simulink model "Mo_phong"  (R2016a)
settings: Solver=ode5  SolverMode=SingleTasking  StartTime=0.0  StopTime=9  FixedStep=0.001  RelTol=1e-3
libraries: simulink x5
settings Model: Creator=nguye  LastModifiedBy=nguye
settings DebuggingCC: SFUnexpectedBacktrackingDiag=error  SFNoUnconditionalDefaultTransitionDiag=error
settings SFSimCC: SimUseLocalCustomCode=on
settings RTWCC: RTWUseLocalCustomCode=on
settings GRTTargetCC: TargetLangStandard=C99 (ISO)  GeneratePreprocessorConditionals=Use local settings
settings ConfigComp: CovMetricSettings=dwe  CovHtmlReporting=off  CovSaveCumulativeToWorkspaceVar=off  CovSaveSingleToWorkspaceVar=off  CovExternalEMLEnable=on

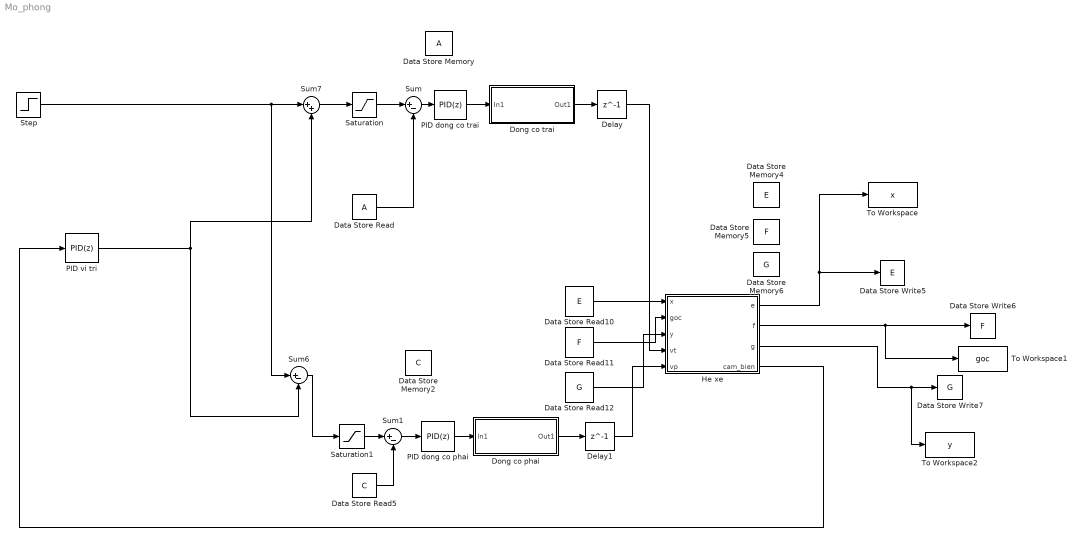
== system Mo_phong ==
  Data Store Memory : DataStoreMemory  ReadBeforeWriteMsg=warning  WriteAfterWriteMsg=warning  WriteAfterReadMsg=warning  ShowAdditionalParam=off
  Data Store Memory2 : DataStoreMemory  DataStoreName=C  ReadBeforeWriteMsg=warning  WriteAfterWriteMsg=warning  WriteAfterReadMsg=warning  ShowAdditionalParam=off
  Data Store Memory4 : DataStoreMemory  DataStoreName=E  ReadBeforeWriteMsg=warning  WriteAfterWriteMsg=warning  WriteAfterReadMsg=warning  ShowAdditionalParam=off
  Data Store Memory5 : DataStoreMemory  DataStoreName=F  ReadBeforeWriteMsg=warning  WriteAfterWriteMsg=warning  WriteAfterReadMsg=warning  ShowAdditionalParam=off
  Data Store Memory6 : DataStoreMemory  DataStoreName=G  ReadBeforeWriteMsg=warning  WriteAfterWriteMsg=warning  WriteAfterReadMsg=warning  ShowAdditionalParam=off
  Data Store Read : DataStoreRead
  Data Store Read10 : DataStoreRead  DataStoreName=E
  Data Store Read11 : DataStoreRead  DataStoreName=F
  Data Store Read12 : DataStoreRead  DataStoreName=G
  Data Store Read5 : DataStoreRead  DataStoreName=C
  Data Store Write5 : DataStoreWrite  DataStoreName=E
  Data Store Write6 : DataStoreWrite  DataStoreName=F
  Data Store Write7 : DataStoreWrite  DataStoreName=G
  Delay : Delay  DelayLength=1  InitialCondition=0
  Delay1 : Delay  DelayLength=1  InitialCondition=0
  Dong co phai : Subsystem
  Dong co trai : Subsystem
  He xe : MATLAB Function  TreatAsAtomicUnit=on
  PID dong co phai : simulink/Continuous/PID Controller  Controller=PID  Form=Parallel  TimeDomain=Discrete-time  SampleTime=0.001  IntegratorMethod=Forward Euler  FilterMethod=Forward Euler  ControllerParametersSource=internal  P=0.25  I=8  D=0.0  UseFilter=off  N=0.08  InitialConditionSource=internal  InitialConditionForIntegrator=0  InitialConditionForFilter=0  DifferentiatorICPrevScaledInput=0  ExternalReset=none  TrackingMode=off  Kt=1  LimitOutput=on  UpperSaturationLimit=100  LowerSaturationLimit=-100  LinearizeAsGain=off  AntiWindupMode=none  Kb=1  POutMin=[]  POutMax=[]  IOutMin=[]  IOutMax=[]  DOutMin=[]  DOutMax=[]  NOutMin=[]  NOutMax=[]  SumOutMin=[]  SumOutMax=[]  SaturationOutMin=[]  SaturationOutMax=[]  PParamMin=[]  PParamMax=[]  IParamMin=[]  IParamMax=[]  DParamMin=[]  DParamMax=[]  NParamMin=[]  NParamMax=[]  KbParamMin=[]  KbParamMax=[]  KtParamMin=[]  KtParamMax=[]  KbOutMin=[]  KbOutMax=[]  KtOutMin=[]  KtOutMax=[]  IntegratorOutMin=[]  IntegratorOutMax=[]  FilterOutMin=[]  FilterOutMax=[]  SumI1OutMin=[]  SumI1OutMax=[]  SumI2OutMin=[]  SumI2OutMax=[]  SumI3OutMin=[]  SumI3OutMax=[]  SumDOutMin=[]  SumDOutMax=[]  DifferentiatorOutMin=[]  DifferentiatorOutMax=[]  IntegratorContinuousStateAttributes=''  IntegratorStateMustResolveToSignalObject=off  IntegratorRTWStateStorageClass=Auto  FilterContinuousStateAttributes=''  FilterStateMustResolveToSignalObject=off  FilterRTWStateStorageClass=Auto
  PID dong co trai : simulink/Continuous/PID Controller  Controller=PID  Form=Parallel  TimeDomain=Discrete-time  SampleTime=0.001  IntegratorMethod=Forward Euler  FilterMethod=Forward Euler  ControllerParametersSource=internal  P=0.25  I=7.5  D=0.0  UseFilter=off  N=0.08  InitialConditionSource=internal  InitialConditionForIntegrator=0  InitialConditionForFilter=0  DifferentiatorICPrevScaledInput=0  ExternalReset=none  TrackingMode=off  Kt=1  LimitOutput=on  UpperSaturationLimit=100  LowerSaturationLimit=-100  LinearizeAsGain=off  AntiWindupMode=none  Kb=1  POutMin=[]  POutMax=[]  IOutMin=[]  IOutMax=[]  DOutMin=[]  DOutMax=[]  NOutMin=[]  NOutMax=[]  SumOutMin=[]  SumOutMax=[]  SaturationOutMin=[]  SaturationOutMax=[]  PParamMin=[]  PParamMax=[]  IParamMin=[]  IParamMax=[]  DParamMin=[]  DParamMax=[]  NParamMin=[]  NParamMax=[]  KbParamMin=[]  KbParamMax=[]  KtParamMin=[]  KtParamMax=[]  KbOutMin=[]  KbOutMax=[]  KtOutMin=[]  KtOutMax=[]  IntegratorOutMin=[]  IntegratorOutMax=[]  FilterOutMin=[]  FilterOutMax=[]  SumI1OutMin=[]  SumI1OutMax=[]  SumI2OutMin=[]  SumI2OutMax=[]  SumI3OutMin=[]  SumI3OutMax=[]  SumDOutMin=[]  SumDOutMax=[]  DifferentiatorOutMin=[]  DifferentiatorOutMax=[]  IntegratorContinuousStateAttributes=''  IntegratorStateMustResolveToSignalObject=off  IntegratorRTWStateStorageClass=Auto  FilterContinuousStateAttributes=''  FilterStateMustResolveToSignalObject=off  FilterRTWStateStorageClass=Auto
  PID vi tri : simulink/Continuous/PID Controller  Controller=PID  Form=Parallel  TimeDomain=Discrete-time  SampleTime=-1  IntegratorMethod=Forward Euler  FilterMethod=Forward Euler  ControllerParametersSource=internal  P=10  I=0  D=2  UseFilter=on  N=1  InitialConditionSource=internal  InitialConditionForIntegrator=0  InitialConditionForFilter=0  DifferentiatorICPrevScaledInput=0  ExternalReset=none  TrackingMode=off  Kt=1  LimitOutput=off  UpperSaturationLimit=inf  LowerSaturationLimit=-inf  LinearizeAsGain=off  AntiWindupMode=none  Kb=1  POutMin=[]  POutMax=[]  IOutMin=[]  IOutMax=[]  DOutMin=[]  DOutMax=[]  NOutMin=[]  NOutMax=[]  SumOutMin=[]  SumOutMax=[]  SaturationOutMin=[]  SaturationOutMax=[]  PParamMin=[]  PParamMax=[]  IParamMin=[]  IParamMax=[]  DParamMin=[]  DParamMax=[]  NParamMin=[]  NParamMax=[]  KbParamMin=[]  KbParamMax=[]  KtParamMin=[]  KtParamMax=[]  KbOutMin=[]  KbOutMax=[]  KtOutMin=[]  KtOutMax=[]  IntegratorOutMin=[]  IntegratorOutMax=[]  FilterOutMin=[]  FilterOutMax=[]  SumI1OutMin=[]  SumI1OutMax=[]  SumI2OutMin=[]  SumI2OutMax=[]  SumI3OutMin=[]  SumI3OutMax=[]  SumDOutMin=[]  SumDOutMax=[]  DifferentiatorOutMin=[]  DifferentiatorOutMax=[]  IntegratorContinuousStateAttributes=''  IntegratorStateMustResolveToSignalObject=off  IntegratorRTWStateStorageClass=Auto  FilterContinuousStateAttributes=''  FilterStateMustResolveToSignalObject=off  FilterRTWStateStorageClass=Auto
  Saturation : Saturate  UpperLimit=292  LowerLimit=25
  Saturation1 : Saturate  UpperLimit=258  LowerLimit=25
  Step : Step  Time=0  After=100
  Sum : Sum  Inputs=|+-
  Sum1 : Sum  Inputs=|+-
  Sum6 : Sum  Inputs=|+-
  Sum7 : Sum  Inputs=|++
  To Workspace : ToWorkspace  VariableName=x  SampleTime=-1
      settings: Save2DSignal=2-D array (concatenate along first dimension)
  To Workspace1 : ToWorkspace  VariableName=goc  SampleTime=-1
      settings: Save2DSignal=2-D array (concatenate along first dimension)
  To Workspace2 : ToWorkspace  VariableName=y  SampleTime=-1
      settings: Save2DSignal=2-D array (concatenate along first dimension)
  wires:
  Step/1 -> Sum6/1, Sum7/1
  Data Store Read/1 -> Sum/2
  Sum/1 -> PID dong co trai/1
  Sum1/1 -> PID dong co phai/1
  Data Store Read5/1 -> Sum1/2
  Sum6/1 -> Saturation1/1
  Sum7/1 -> Saturation/1
  Saturation/1 -> Sum/1
  Saturation1/1 -> Sum1/1
  Delay/1 -> He xe/4(vt)
  Delay1/1 -> He xe/5(vp)
  Data Store Read10/1 -> He xe/1(x)
  Data Store Read11/1 -> He xe/2(goc)
  Data Store Read12/1 -> He xe/3(y)
  He xe/1(e) -> To Workspace/1, Data Store Write5/1
  He xe/2(f) -> Data Store Write6/1, To Workspace1/1
  He xe/3(g) -> Data Store Write7/1, To Workspace2/1
  He xe/4(cam_bien) -> PID vi tri/1
  PID vi tri/1 -> Sum7/2, Sum6/2
  PID dong co trai/1 -> Dong co trai/1(In1)
  Dong co trai/1(Out1) -> Delay/1
  PID dong co phai/1 -> Dong co phai/1(In1)
  Dong co phai/1(Out1) -> Delay1/1

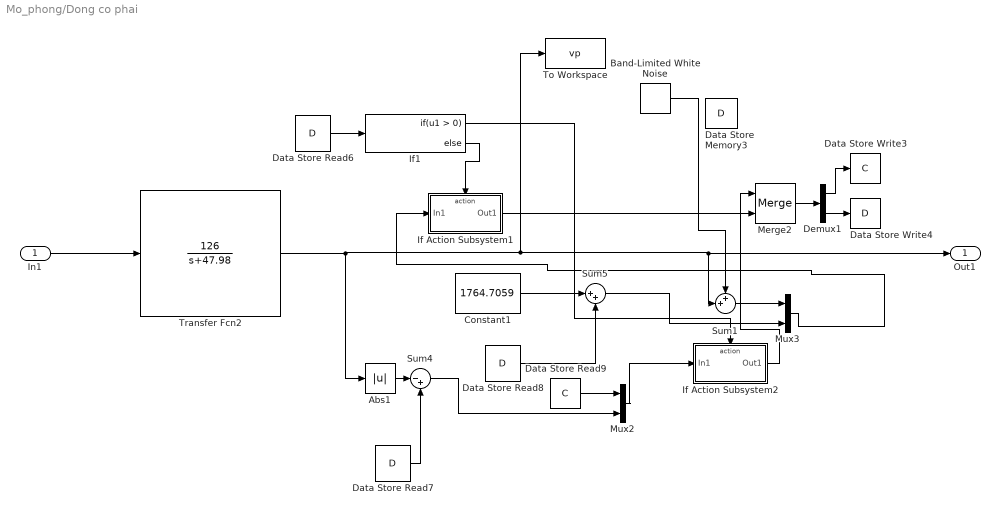
== system Mo_phong/Dong co phai ==
  In1 : Inport
  Abs1 : Abs
  Band-Limited White Noise : simulink/Sources/Band-Limited White Noise  Cov=[0.005]  Ts=0.001  seed=[23341]
  Constant1 : Constant  Value=1764.7059
  Data Store Memory3 : DataStoreMemory  DataStoreName=D  ReadBeforeWriteMsg=warning  WriteAfterWriteMsg=warning  WriteAfterReadMsg=warning  InitialValue=1764.7059  ShowAdditionalParam=off
  Data Store Read6 : DataStoreRead  DataStoreName=D
  Data Store Read7 : DataStoreRead  DataStoreName=D
  Data Store Read8 : DataStoreRead  DataStoreName=D
  Data Store Read9 : DataStoreRead  DataStoreName=C
  Data Store Write3 : DataStoreWrite  DataStoreName=C
  Data Store Write4 : DataStoreWrite  DataStoreName=D
  Demux1 : Demux  Outputs=2
  If Action Subsystem1 : Subsystem  TreatAsAtomicUnit=on
  If Action Subsystem2 : Subsystem  TreatAsAtomicUnit=on
  If1 : If
  Merge2 : Merge
  Mux2 : Mux  Inputs=2
  Mux3 : Mux  Inputs=2
  Sum1 : Sum  Inputs=++|
  Sum4 : Sum  Inputs=|-+
  Sum5 : Sum  Inputs=|++
  To Workspace : ToWorkspace  VariableName=vp  SampleTime=-1
      settings: Save2DSignal=2-D array (concatenate along first dimension)
  Transfer Fcn2 : TransferFcn  Numerator=[126]  Denominator=[1 47.98]
  Out1 : Outport
  wires:
  Sum4/1 -> Mux2/2
  Transfer Fcn2/1 -> To Workspace/1, Sum1/2, Out1/1, Abs1/1
  Data Store Read6/1 -> If1/1
  If Action Subsystem1/1(Out1) -> Merge2/2
  Data Store Read8/1 -> Sum5/2
  Data Store Read7/1 -> Sum4/2
  Sum5/1 -> Mux3/2
  If1/1 -> If Action Subsystem2/Action
  Abs1/1 -> Sum4/1
  If1/2 -> If Action Subsystem1/Action
  Constant1/1 -> Sum5/1
  Mux2/1 -> If Action Subsystem2/1(In1)
  Demux1/2 -> Data Store Write4/1
  Mux3/1 -> If Action Subsystem1/1(In1)
  In1/1 -> Transfer Fcn2/1
  Data Store Read9/1 -> Mux2/1
  Merge2/1 -> Demux1/1
  If Action Subsystem2/1(Out1) -> Merge2/1
  Demux1/1 -> Data Store Write3/1
  Sum1/1 -> Mux3/1
  Band-Limited White Noise/1 -> Sum1/1

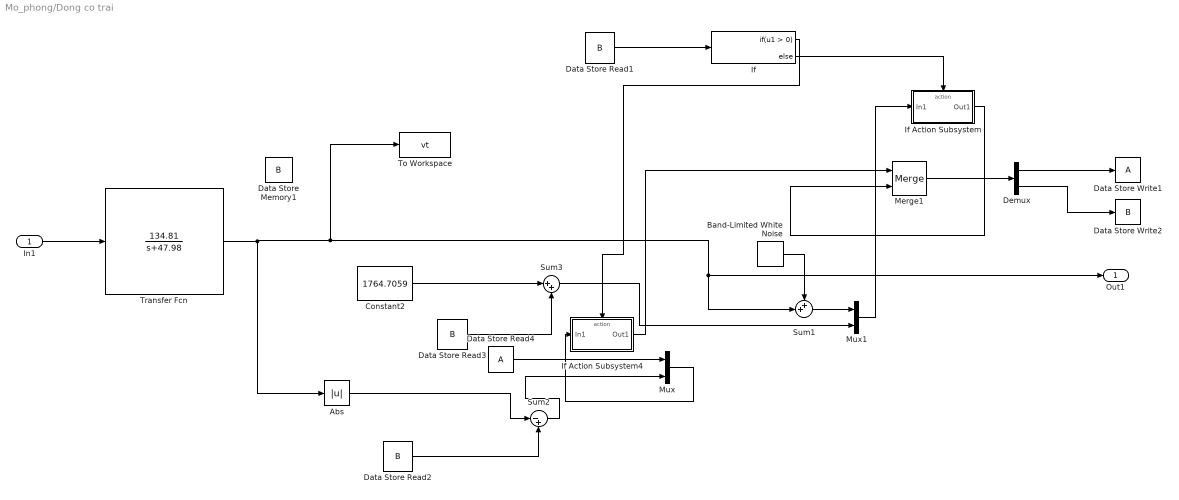
== system Mo_phong/Dong co trai ==
  In1 : Inport
  Abs : Abs
  Band-Limited White Noise : simulink/Sources/Band-Limited White Noise  Cov=[0.005]  Ts=0.001  seed=[23341]
  Constant2 : Constant  Value=1764.7059
  Data Store Memory1 : DataStoreMemory  DataStoreName=B  ReadBeforeWriteMsg=warning  WriteAfterWriteMsg=warning  WriteAfterReadMsg=warning  InitialValue=1764.7059  ShowAdditionalParam=off
  Data Store Read1 : DataStoreRead  DataStoreName=B
  Data Store Read2 : DataStoreRead  DataStoreName=B
  Data Store Read3 : DataStoreRead  DataStoreName=B
  Data Store Read4 : DataStoreRead
  Data Store Write1 : DataStoreWrite
  Data Store Write2 : DataStoreWrite  DataStoreName=B
  Demux : Demux  Outputs=2
  If : If
  If Action Subsystem : Subsystem  TreatAsAtomicUnit=on
  If Action Subsystem4 : Subsystem  TreatAsAtomicUnit=on
  Merge1 : Merge
  Mux : Mux  Inputs=2
  Mux1 : Mux  Inputs=2
  Sum1 : Sum  Inputs=++|
  Sum2 : Sum  Inputs=|-+
  Sum3 : Sum  Inputs=|++
  To Workspace : ToWorkspace  VariableName=vt  SampleTime=-1
      settings: Save2DSignal=2-D array (concatenate along first dimension)
  Transfer Fcn : TransferFcn  Numerator=[134.81]  Denominator=[1 47.98]
  Out1 : Outport
  wires:
  Data Store Read2/1 -> Sum2/2
  Merge1/1 -> Demux/1
  Data Store Read3/1 -> Sum3/2
  Mux1/1 -> If Action Subsystem/1(In1)
  Abs/1 -> Sum2/1
  Constant2/1 -> Sum3/1
  Data Store Read4/1 -> Mux/1
  Demux/1 -> Data Store Write1/1
  Demux/2 -> Data Store Write2/1
  Data Store Read1/1 -> If/1
  If/1 -> If Action Subsystem4/Action
  If Action Subsystem4/1(Out1) -> Merge1/1
  Mux/1 -> If Action Subsystem4/1(In1)
  In1/1 -> Transfer Fcn/1
  Sum3/1 -> Mux1/2
  If Action Subsystem/1(Out1) -> Merge1/2
  Transfer Fcn/1 -> To Workspace/1, Sum1/2, Out1/1, Abs/1
  Sum2/1 -> Mux/2
  If/2 -> If Action Subsystem/Action
  Sum1/1 -> Mux1/1
  Band-Limited White Noise/1 -> Sum1/1

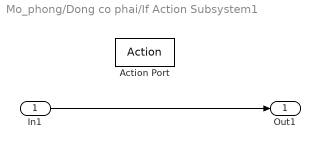
== system Mo_phong/Dong co phai/If Action Subsystem1 ==
  In1 : Inport
  Action Port : ActionPort  ActionType=else
  Out1 : Outport
  wires:
  In1/1 -> Out1/1

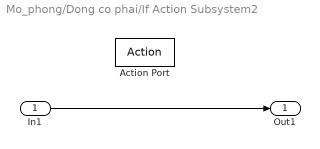
== system Mo_phong/Dong co phai/If Action Subsystem2 ==
  In1 : Inport
  Action Port : ActionPort  ActionType=then
  Out1 : Outport
  wires:
  In1/1 -> Out1/1

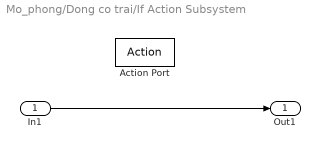
== system Mo_phong/Dong co trai/If Action Subsystem ==
  In1 : Inport
  Action Port : ActionPort  ActionType=else
  Out1 : Outport
  wires:
  In1/1 -> Out1/1

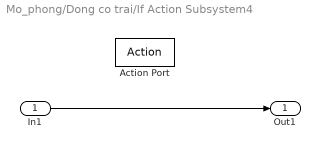
== system Mo_phong/Dong co trai/If Action Subsystem4 ==
  In1 : Inport
  Action Port : ActionPort  ActionType=then
  Out1 : Outport
  wires:
  In1/1 -> Out1/1

== matlab function Mo_phong/He xe ==
  data: x input; e output; goc input; y input; vt input; vp input; f output; g output; cam_bien output
function [e,f,g,cam_bien] = fcn(x,goc,y,vt,vp)
v=(vt+vp)*0.065*pi/120;
f=goc+0.001*(vt-vp)*0.065*pi/0.178/60;
e=x+v*sin(f)*0.001;
g=y+v*cos(f)*0.001;
x_dau=e+0.2395*sin(f);
y_dau=g+0.2395*cos(f);
a=0;
a=[0];
b=y_dau+tan(f)*x_dau;
if(b(1)>1.5)
a=double(fzero(@(x)1.5+0.5-0.5/5^(6*x)+tan(f)*x-y_dau-tan(f)*x_dau,0));
b=1.5+0.5-0.5/5^(6*a);
end
u=[a-e b-g 0];
v=[x_dau-e y_dau-g 0];
t=cross(v,u);
toa_do=sign(t(3))*sqrt((a(1)-x_dau)^2+(b(1)-y_dau)^2);
if(toa_do<=0.0085) && (toa_do>=-0.0085)
    cam_bien=0;
elseif(toa_do>=-0.0255)&&(toa_do<-0.0085)
    cam_bien=1;
elseif(toa_do>=-0.0425)&&(toa_do<-0.0255)
    cam_bien=2;
elseif(toa_do<-0.0425)
    cam_bien=3;
elseif(toa_do<=0.0255)&&(toa_do>0.0085)
    cam_bien=-1;
elseif(toa_do<=0.0425)&&(toa_do>0.0255)
    cam_bien=-2;
else(toa_do>0.0425)
    cam_bien=-3;
end
end
